simulink model "SS_eig_LQR"  (R2021a)
settings: Solver=ode45  StartTime=0.0  StopTime=3  RelTol=1e-3
undefined symbols (not defined in the file): daq, der, drv, est_par, gbox, lqr_app_int, mld, mot, nominal, rads2rpm, rpm2rads, sens
settings Model: Creator=gioel  LastModifiedBy=gioel
settings DataIOCC: ReturnWorkspaceOutputs=off

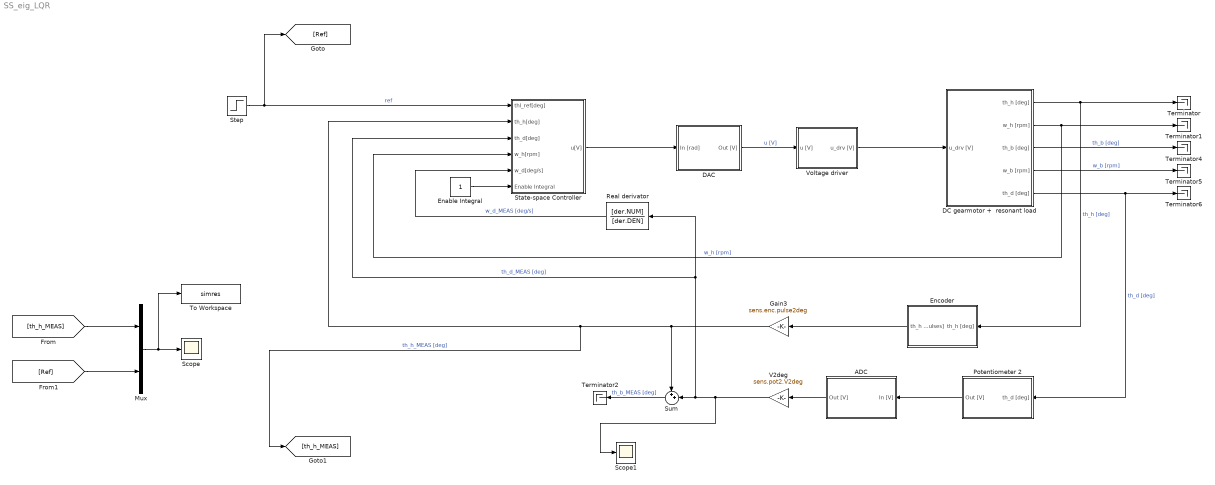
== system SS_eig_LQR ==
  ADC : Subsystem
  DAC : Subsystem
  DC gearmotor +  resonant load : Subsystem
  Enable Integral : Constant
  Encoder : Subsystem
  Gain3 : Gain  Gain=sens.enc.pulse2deg
  Mux : Mux  Inputs=2
  Potentiometer 2 : Subsystem
  Real derivator : TransferFcn  Numerator=[der.NUM]  Denominator=[der.DEN]
  Scope : Scope
  Scope1 : Scope
  State-space Controller : Subsystem
  Step : Step  Time=0  After=50  SampleTime=0
  Sum : Sum  Inputs=++|
  Terminator{,1..2,4..6} (6 alike) : Terminator
  To Workspace : ToWorkspace  VariableName=simres  SaveFormat=Structure With Time  SampleTime=-1
  V2deg : Gain  Gain=sens.pot2.V2deg
  Voltage driver : Subsystem
  wires:
  Encoder/1(th_h [pulses]) -> Gain3/1
  Potentiometer 2/1(Out [V]) -> ADC/1(In [V])
  DC gearmotor +  resonant load/3(th_b [deg]) -> Terminator4/1  "th_b [deg]"
  ADC/1(Out [V]) -> V2deg/1
  V2deg/1 -> Scope1/1, Real derivator/1, State-space Controller/3(th_d[deg]), Sum/2  "th_d_MEAS [deg]"
  State-space Controller/1(u[V]) -> DAC/1(In [rad])
  DC gearmotor +  resonant load/5(th_d [deg]) -> Terminator6/1, Potentiometer 2/1(th_d [deg])  "th_d [deg]"
  DC gearmotor +  resonant load/2(w_h [rpm]) -> State-space Controller/4(w_h[rpm]), Terminator1/1  "w_h [rpm]"
  DAC/1(Out [V]) -> Voltage driver/1(u [V])  "u [V]"
  Gain3/1 -> State-space Controller/2(th_h[deg]), [th_h_MEAS], Sum/1  "th_h_MEAS [deg]"
  DC gearmotor +  resonant load/4(w_b [rpm]) -> Terminator5/1  "w_b [rpm]"
  DC gearmotor +  resonant load/1(th_h [deg]) -> Terminator/1, Encoder/1(th_h [deg])  "th_h [deg]"
  Sum/1 -> Terminator2/1  "th_b_MEAS [deg]"
  Real derivator/1 -> State-space Controller/5(w_d[deg/s])  "w_d_MEAS [deg/s]"
  Step/1 -> State-space Controller/1(thl_ref[deg]), [Ref]  "ref"
  [th_h_MEAS] -> Mux/1
  Mux/1 -> Scope/1, To Workspace/1
  [Ref] -> Mux/2
  Enable Integral/1 -> State-space Controller/6(Enable Integral)
  Voltage driver/1(u_drv [V]) -> DC gearmotor +  resonant load/1(u_drv [V])

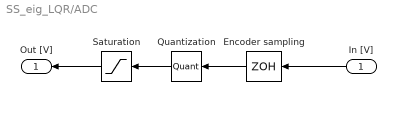
== system SS_eig_LQR/ADC ==
  In [V] : Inport
  Encoder sampling : ZeroOrderHold  SampleTime=sens.enc.T_s
  Quantization : Quantizer  QuantizationInterval=daq.adc.q
  Saturation : Saturate  UpperLimit=daq.adc.fs  LowerLimit=-daq.adc.fs
  Out [V] : Outport
  wires:
  Encoder sampling/1 -> Quantization/1
  Quantization/1 -> Saturation/1
  In [V]/1 -> Encoder sampling/1
  Saturation/1 -> Out [V]/1

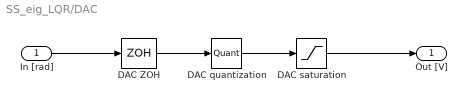
== system SS_eig_LQR/DAC ==
  In [rad] : Inport
  DAC ZOH : ZeroOrderHold  SampleTime=sens.enc.T_s
  DAC quantization : Quantizer  QuantizationInterval=daq.dac.q
  DAC saturation : Saturate  UpperLimit=daq.dac.vdd  LowerLimit=daq.dac.vss
  Out [V] : Outport
  wires:
  DAC quantization/1 -> DAC saturation/1
  DAC ZOH/1 -> DAC quantization/1
  DAC saturation/1 -> Out [V]/1
  In [rad]/1 -> DAC ZOH/1

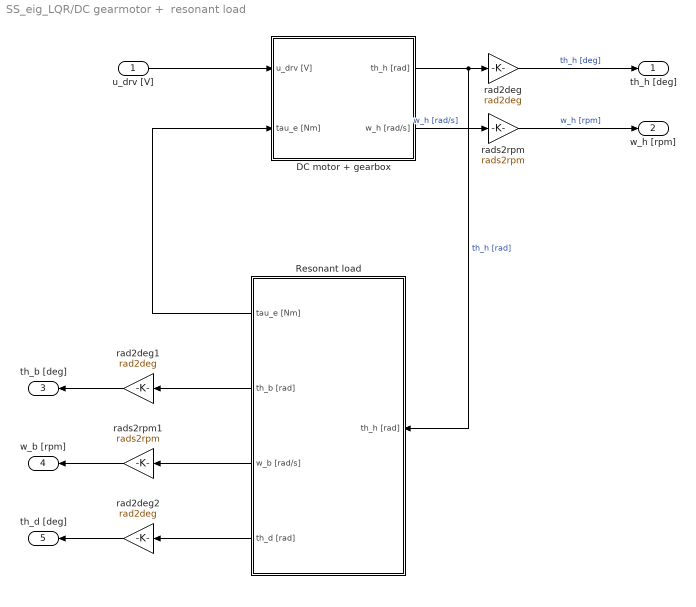
== system SS_eig_LQR/DC gearmotor +  resonant load ==
  u_drv [V] : Inport
  DC motor + gearbox : Subsystem
  Resonant load : Subsystem
  rad2deg : Gain  Gain=rad2deg
  rad2deg1 : Gain  Gain=rad2deg
  rad2deg2 : Gain  Gain=rad2deg
  rads2rpm : Gain  Gain=rads2rpm
  rads2rpm1 : Gain  Gain=rads2rpm
  th_h [deg] : Outport
  w_h [rpm] : Outport  Port=2
  th_b [deg] : Outport  Port=3
  w_b [rpm] : Outport  Port=4
  th_d [deg] : Outport  Port=5
  wires:
  rads2rpm1/1 -> w_b [rpm]/1
  DC motor + gearbox/2(w_h [rad/s]) -> rads2rpm/1  "w_h [rad/s]"
  rad2deg1/1 -> th_b [deg]/1
  u_drv [V]/1 -> DC motor + gearbox/1(u_drv [V])
  Resonant load/3(w_b [rad/s]) -> rads2rpm1/1
  rad2deg2/1 -> th_d [deg]/1
  Resonant load/4(th_d [rad]) -> rad2deg2/1
  Resonant load/2(th_b [rad]) -> rad2deg1/1
  rad2deg/1 -> th_h [deg]/1  "th_h [deg]"
  rads2rpm/1 -> w_h [rpm]/1  "w_h [rpm]"
  DC motor + gearbox/1(th_h [rad]) -> Resonant load/1(th_h [rad]), rad2deg/1  "th_h [rad]"
  Resonant load/1(tau_e [Nm]) -> DC motor + gearbox/2(tau_e [Nm])

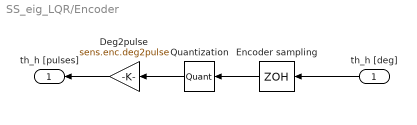
== system SS_eig_LQR/Encoder ==
  th_h [deg] : Inport
  Deg2pulse : Gain  Gain=sens.enc.deg2pulse
  Encoder sampling : ZeroOrderHold  SampleTime=sens.enc.T_s
  Quantization : Quantizer  QuantizationInterval=sens.enc.q
  th_h [pulses] : Outport
  wires:
  Encoder sampling/1 -> Quantization/1
  Quantization/1 -> Deg2pulse/1
  th_h [deg]/1 -> Encoder sampling/1
  Deg2pulse/1 -> th_h [pulses]/1

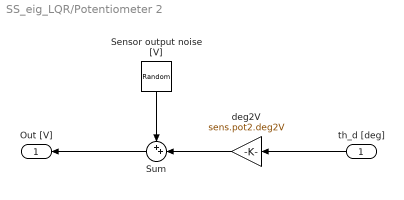
== system SS_eig_LQR/Potentiometer 2 ==
  th_d [deg] : Inport
  Sensor output noise [V] : RandomNumber  Variance=sens.pot2.noise.var  SampleTime=0.1
  Sum : Sum  Inputs=++|
  deg2V : Gain  Gain=sens.pot2.deg2V
  Out [V] : Outport
  wires:
  Sum/1 -> Out [V]/1
  th_d [deg]/1 -> deg2V/1
  deg2V/1 -> Sum/2
  Sensor output noise [V]/1 -> Sum/1

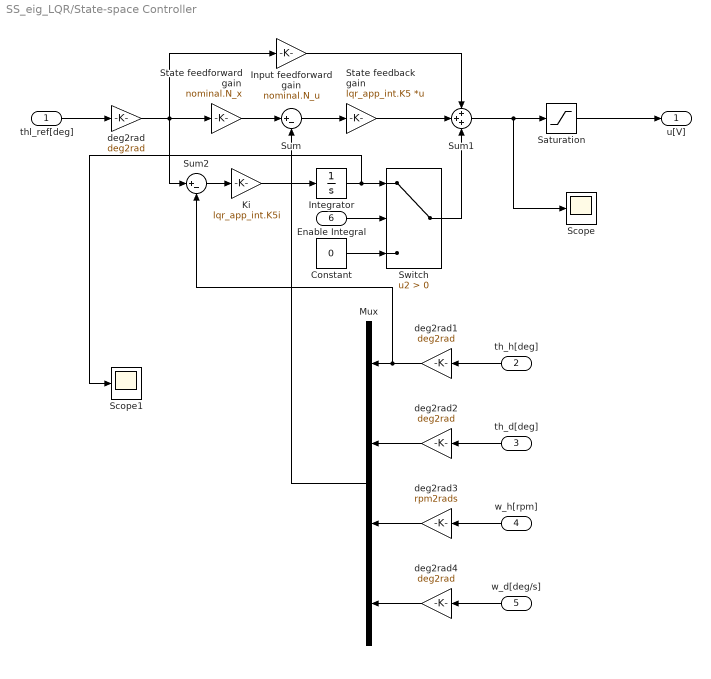
== system SS_eig_LQR/State-space Controller ==
  thl_ref[deg] : Inport
  th_h[deg] : Inport  Port=2
  th_d[deg] : Inport  Port=3
  w_h[rpm] : Inport  Port=4
  w_d[deg/s] : Inport  Port=5
  Enable Integral : Inport  Port=6
  Constant : Constant  Value=0
  Input feedforward gain : Gain  Gain=nominal.N_u
  Integrator : Integrator
  Ki : Gain  Gain=lqr_app_int.K5i
  Mux : Mux
  Saturation : Saturate  UpperLimit=10  LowerLimit=-10
  Scope : Scope
  Scope1 : Scope
  State feedback gain : Gain  Gain=lqr_app_int.K5  Multiplication=Matrix(K*u)
  State feedforward gain : Gain  Gain=nominal.N_x
  Sum : Sum  Inputs=|+-
  Sum1 : Sum  Inputs=+++
  Sum2 : Sum  Inputs=|+-
  Switch : Switch  Criteria=u2 > Threshold
  deg2rad{,1..2,4} (4 alike) : Gain  Gain=deg2rad
  deg2rad3 : Gain  Gain=rpm2rads
  u[V] : Outport
  wires:
  thl_ref[deg]/1 -> deg2rad/1
  deg2rad/1 -> Sum2/1, Input feedforward gain/1, State feedforward gain/1
  th_h[deg]/1 -> deg2rad1/1
  Saturation/1 -> u[V]/1
  State feedforward gain/1 -> Sum/1
  Sum/1 -> State feedback gain/1
  Mux/1 -> Sum/2
  Sum1/1 -> Scope/1, Saturation/1
  Input feedforward gain/1 -> Sum1/1
  State feedback gain/1 -> Sum1/2
  Sum2/1 -> Ki/1
  deg2rad1/1 -> Sum2/2, Mux/1
  Ki/1 -> Integrator/1
  Switch/1 -> Sum1/3
  Integrator/1 -> Scope1/1, Switch/1
  th_d[deg]/1 -> deg2rad2/1
  w_d[deg/s]/1 -> deg2rad4/1
  deg2rad2/1 -> Mux/2
  w_h[rpm]/1 -> deg2rad3/1
  deg2rad3/1 -> Mux/3
  deg2rad4/1 -> Mux/4
  Constant/1 -> Switch/3
  Enable Integral/1 -> Switch/2

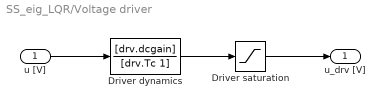
== system SS_eig_LQR/Voltage driver ==
  u [V] : Inport
  Driver dynamics : TransferFcn  Numerator=[drv.dcgain]  Denominator=[drv.Tc 1]
  Driver saturation : Saturate  UpperLimit=drv.outmax  LowerLimit=-drv.outmax
  u_drv [V] : Outport
  wires:
  Driver saturation/1 -> u_drv [V]/1
  Driver dynamics/1 -> Driver saturation/1
  u [V]/1 -> Driver dynamics/1

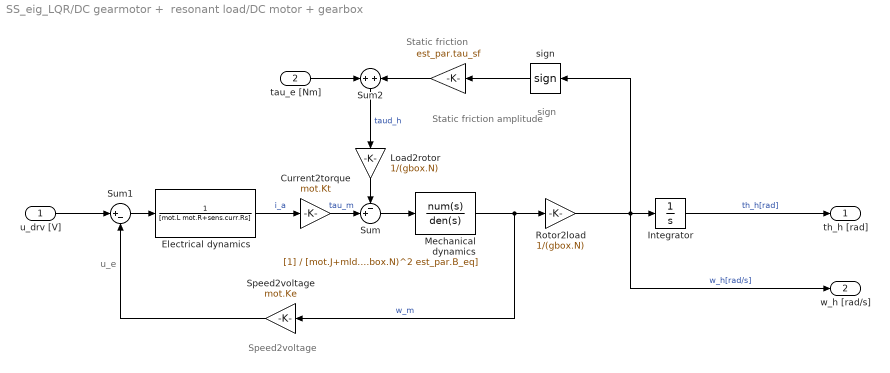
== system SS_eig_LQR/DC gearmotor +  resonant load/DC motor + gearbox ==
  note: u_e
  note: Speed2voltage
  note: Static friction
  note: sign
  note: Static friction
      |  amplitude
  u_drv [V] : Inport
  tau_e [Nm] : Inport  Port=2
  " " : Gain  Gain=est_par.tau_sf
  Current2torque : Gain  Gain=mot.Kt
  Electrical dynamics : TransferFcn  Denominator=[mot.L mot.R+sens.curr.Rs]
  Integrator : Integrator
  Load2rotor : Gain  Gain=1/(gbox.N)
  Mechanical dynamics : TransferFcn  Denominator=[mot.J+mld.Jh/(gbox.N)^2 est_par.B_eq]
  Rotor2load : Gain  Gain=1/(gbox.N)
  Speed2voltage : Gain  Gain=mot.Ke
  Sum : Sum  Inputs=-+|
  Sum1 : Sum  Inputs=|+-
  Sum2 : Sum  Inputs=+|+
  sign : Signum  ZeroCross=off
  th_h [rad] : Outport
  w_h [rad/s] : Outport  Port=2
  wires:
  u_drv [V]/1 -> Sum1/1
  Electrical dynamics/1 -> Current2torque/1  "i_a"
  Current2torque/1 -> Sum/2  "tau_m"
  sign/1 -> " "/1
  Sum1/1 -> Electrical dynamics/1
  Integrator/1 -> th_h [rad]/1  "th_h[rad]"
  Sum/1 -> Mechanical dynamics/1
  Load2rotor/1 -> Sum/1
  Speed2voltage/1 -> Sum1/2
  Rotor2load/1 -> w_h [rad/s]/1, sign/1, Integrator/1  "w_h[rad/s]"
  Mechanical dynamics/1 -> Speed2voltage/1, Rotor2load/1  "w_m"
  " "/1 -> Sum2/2
  Sum2/1 -> Load2rotor/1  "taud_h"
  tau_e [Nm]/1 -> Sum2/1

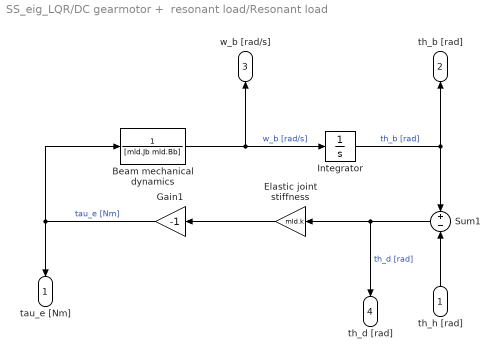
== system SS_eig_LQR/DC gearmotor +  resonant load/Resonant load ==
  th_h [rad] : Inport
  Beam mechanical dynamics : TransferFcn  Denominator=[mld.Jb mld.Bb]
  Elastic joint stiffness : Gain  Gain=mld.k
  Gain1 : Gain  Gain=-1
  Integrator : Integrator
  Sum1 : Sum  Inputs=+|-
  tau_e [Nm] : Outport
  th_b [rad] : Outport  Port=2
  w_b [rad/s] : Outport  Port=3
  th_d [rad] : Outport  Port=4
  wires:
  th_h [rad]/1 -> Sum1/2
  Gain1/1 -> tau_e [Nm]/1, Beam mechanical dynamics/1  "tau_e [Nm]"
  Elastic joint stiffness/1 -> Gain1/1
  Sum1/1 -> th_d [rad]/1, Elastic joint stiffness/1  "th_d [rad]"
  Integrator/1 -> th_b [rad]/1, Sum1/1  "th_b [rad]"
  Beam mechanical dynamics/1 -> w_b [rad/s]/1, Integrator/1  "w_b [rad/s]"
